simulink subsystem "attitude_control"  (R2024a)
settings: Solver=VariableStepAuto  StartTime=0.0  StopTime=10.0  RelTol=1e-3
libraries: matrix_library x2, aerolibutil x2
settings Model: Creator=joshu  LastModifiedBy=joshu

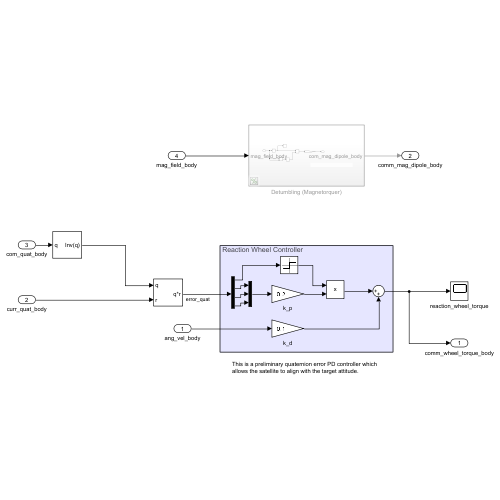
[thumbnail: Simulink's stored preview of the top-level diagram]
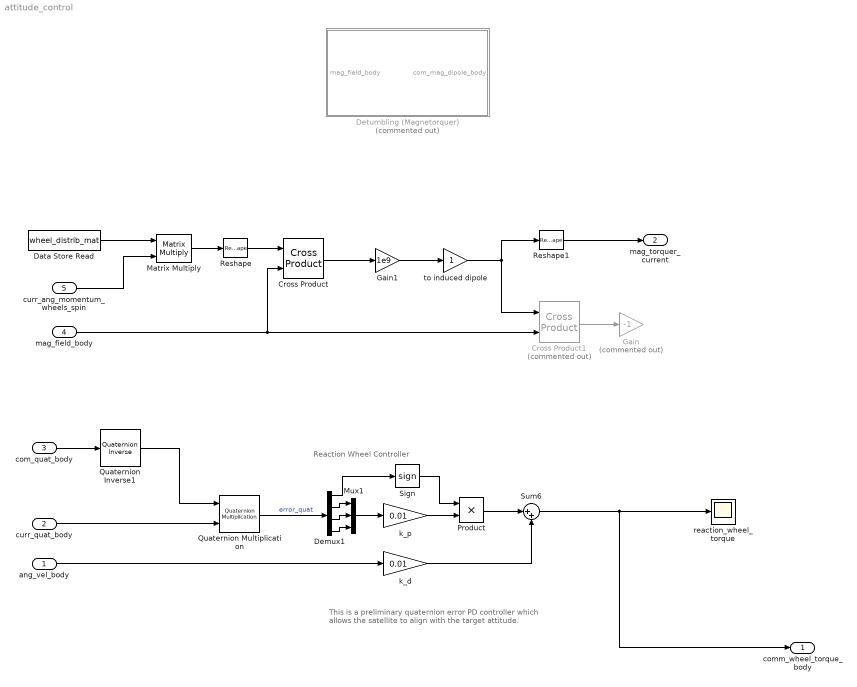
== system attitude_control ==
  note: This is a preliminary quaternion error PD controller which allows the satellite to align with the target attitude.
  note: Reaction Wheel Controller
  ang_vel_body : Inport
  curr_quat_body : Inport  Port=2
  com_quat_body : Inport  Port=3
  mag_field_body : Inport  Port=4
  curr_ang_momentum_wheels_spin : Inport  Port=5
  Cross Product : matrix_library/Cross Product
  Cross Product1 : matrix_library/Cross Product  Commented=on
  Data Store Read : DataStoreRead  DataStoreName=wheel_distrib_mat  IndexOptions=Index vector (dialog)  Indices=1  OutputSizes=1
  Demux1 : Demux
  Detumbling (Magnetorquer) : Subsystem  Commented=on
  Gain : Gain  Commented=on  Gain=-1
  Gain1 : Gain  Gain=1e9
  Matrix Multiply : Product  Multiplication=Matrix(*)
  Mux1 : Mux  Inputs=3
  Product : Product
  Quaternion Inverse1 : aerolibutil/Quaternion Inverse
  Quaternion Multiplication : aerolibutil/Quaternion Multiplication
  Reshape : Reshape  OutputDimensionality=Row vector (2-D)
  Reshape1 : Reshape
  Sign : Signum
  Sum6 : Sum  Inputs=|++
  k_d : Gain  Gain=0.01
  k_p : Gain  Gain=0.01
  reaction_wheel_torque : Scope
  to induced dipole : Gain
  comm_wheel_torque_body : Outport
  mag_torquer_current : Outport  Port=2
  wires:
  k_d/1 -> Sum6/2
  com_quat_body/1 -> Quaternion Inverse1/1
  Demux1/2 -> Mux1/1
  ang_vel_body/1 -> k_d/1
  Sum6/1 -> reaction_wheel_torque/1, comm_wheel_torque_body/1
  curr_quat_body/1 -> Quaternion Multiplication/2
  Quaternion Multiplication/1 -> Demux1/1  "error_quat"
  Demux1/1 -> Sign/1
  Product/1 -> Sum6/1
  k_p/1 -> Product/2
  Quaternion Inverse1/1 -> Quaternion Multiplication/1
  Mux1/1 -> k_p/1
  Sign/1 -> Product/1
  Demux1/4 -> Mux1/3
  Demux1/3 -> Mux1/2
  Cross Product1/1 -> Gain/1
  Cross Product/1 -> Gain1/1
  Data Store Read/1 -> Matrix Multiply/1
  curr_ang_momentum_wheels_spin/1 -> Matrix Multiply/2
  mag_field_body/1 -> Cross Product/2, Cross Product1/2
  to induced dipole/1 -> Cross Product1/1, Reshape1/1
  Matrix Multiply/1 -> Reshape/1
  Reshape/1 -> Cross Product/1
  Gain1/1 -> to induced dipole/1
  Reshape1/1 -> mag_torquer_current/1

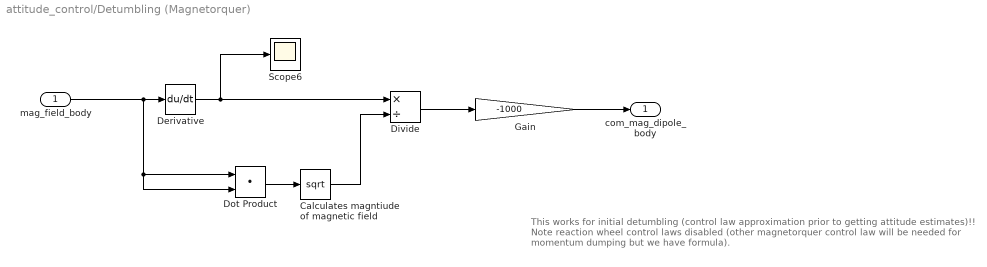
== system attitude_control/Detumbling (Magnetorquer) ==
  note: This works for initial detumbling (control law approximation prior to getting attitude estimates)!! Note reaction wheel control laws disabled (other magnetorquer control law will be needed for momentum dumping but we have formula).
  mag_field_body : Inport
  Calculates magntiude of magnetic field : Sqrt
  Derivative : Derivative
  Divide : Product  Inputs=*/
  Dot Product : DotProduct  OutDataTypeStr=Inherit: Inherit via internal rule
  Gain : Gain  Gain=-1000
  Scope6 : Scope
  com_mag_dipole_body : Outport
  wires:
  Calculates magntiude of magnetic field/1 -> Divide/2
  Gain/1 -> com_mag_dipole_body/1
  Dot Product/1 -> Calculates magntiude of magnetic field/1
  Divide/1 -> Gain/1
  mag_field_body/1 -> Derivative/1, Dot Product/2, Dot Product/1
  Derivative/1 -> Divide/1, Scope6/1
